simulink model "bbsr_sim"  (R2022b)
settings: Solver=VariableStepAuto  StartTime=0.0  StopTime=tmax  MaxStep=dt  RelTol=1e-3
values from neighbouring files (symbols this model uses):
  burning_rate = 1018/32.42    (= 31.4003701419)    [black_brant_vc.m]
  D0 = 1.225    [earth.m]
  fthrust = 69.4*10^3    (= 69400)    [black_brant_vc.m]
  G = 6.67430*10^-11    (= 6.6743e-11)    [bbsr_driverfile.m]
  H = 7640    [earth.m]
  mearth = 5.9722*10^24    (= 5.9722e+24)    [earth.m]
  mfuel = 1018    [black_brant_vc.m]
  mpayload = 100    [black_brant_vc.m]
  mrocket = 1261    [black_brant_vc.m]
  nozzle_area = pi*0.34^2    (= 0.363168110755)    [black_brant_vc.m]
  P0 = 1.01325*10^5    (= 101325)    [earth.m]
  pitch = 60*rad    (= 1.0471975512)    [bbsr_driverfile.m]
  r_earth = 6.3781*10^6    (= 6378100)    [earth.m]
  railheight = sin(pitch)*25    [bbsr_driverfile.m]
  v0 = 0    [bbsr_driverfile.m]
  x0 = 0    [bbsr_driverfile.m]
  y0 = 0    [bbsr_driverfile.m]
libraries: simulink x1
settings Model: Creator=mitch  LastModifiedBy=mitch
settings DataIOCC: ReturnWorkspaceOutputs=off

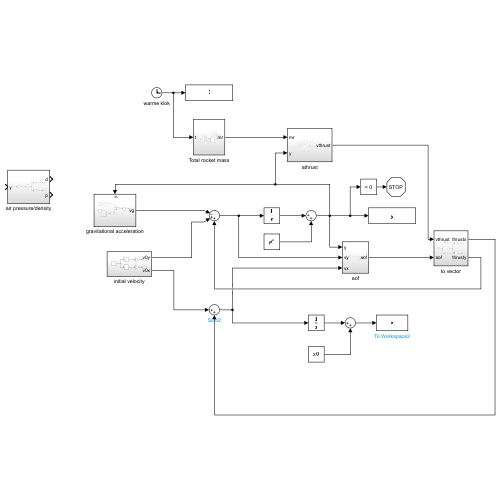
[thumbnail: Simulink's stored preview of the top-level diagram]
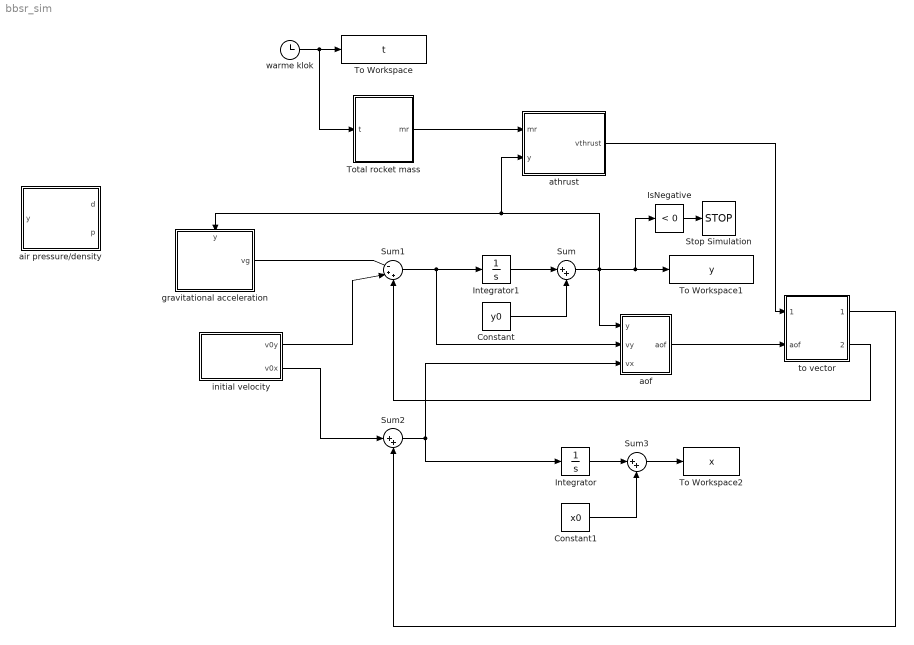
== system bbsr_sim ==
  Constant : Constant  Value=y0
  Constant1 : Constant  Value=x0
  Integrator : Integrator
  Integrator1 : Integrator
  IsNegative : simulink/Logic and Bit Operations/Compare To Zero  relop=<  OutDataTypeStr=boolean
      settings: LibrarySourceBlock=|
      | simulink/Quick Insert/Logic and Bit
      | Operations/IsNegative
  Stop Simulation : Stop
  Sum : Sum  Inputs=|++
  Sum1 : Sum  Inputs=|-++
  Sum2 : Sum  Inputs=|++
  Sum3 : Sum  Inputs=|++
  To Workspace : ToWorkspace  VariableName=t  SampleTime=-1
  To Workspace1 : ToWorkspace  VariableName=y  SampleTime=-1
  To Workspace2 : ToWorkspace  VariableName=x  SampleTime=-1
  Total rocket mass : Subsystem
  air pressure/density : Subsystem
  aof : Subsystem
  athrust : Subsystem
  gravitational acceleration : Subsystem
      settings: PortSchema="{\"entries\":[{\"content\":{\"sides\":[{\"content\":{\"connectorIds\":[]},\"type\":\"ConnectorPlacement.EquallySpacedRectSide\",\"uuid\":\"49ae1f6c-9b05-4d5e-bf5d-de0f817c918d\"},{\"content\":{\"connectorIds\":[\"Out1\"],\"side\":\"RIGHT\"},\"type\":\"ConnectorPlacement.EquallySpacedRectSide\",\"uuid\":\"2668f6bc-3456-4f0e-9125-4666e44a9436\"},{\"content\":{\"connectorIds\":[\"In1\"],\"side\":\"TOP\"},\"type\":\"ConnectorPlacement.EquallySpacedRectSide\",\"uuid\":\"db408307-21fd-484d-89bb-a4b1247c71c3\"}]},\"type\":\"ConnectorPlacement.EquallySpacedConnector\",\"uuid\":\"81d98a46-5b23-44e6-b19a-9d7581a6447a\"}],\"packageUris\":[\"http://schema.mathworks.com/mf0/Connector/R2020b\"],\"version\":\"1.0\"}"
  initial velocity : Subsystem
  to vector : Subsystem
  warme klok : Clock
  wires:
  warme klok/1 -> Total rocket mass/1(t), To Workspace/1
  Total rocket mass/1(mr) -> athrust/1(mr)
  Integrator1/1 -> Sum/1
  Sum/1 -> aof/1(y), athrust/2(y), gravitational acceleration/1(y), IsNegative/1, To Workspace1/1
  Constant/1 -> Sum/2
  gravitational acceleration/1(vg) -> Sum1/1
  Sum1/1 -> aof/2(vy), Integrator1/1
  initial velocity/1(v0y) -> Sum1/2
  athrust/1(vthrust) -> to vector/1(vthrust)
  aof/1(aof) -> to vector/2(aof)
  to vector/2(thrusty) -> Sum1/3
  initial velocity/2(v0x) -> Sum2/1
  to vector/1(thrustx) -> Sum2/2
  Sum2/1 -> aof/3(vx), Integrator/1
  Integrator/1 -> Sum3/1
  Sum3/1 -> To Workspace2/1
  Constant1/1 -> Sum3/2
  IsNegative/1 -> Stop Simulation/1

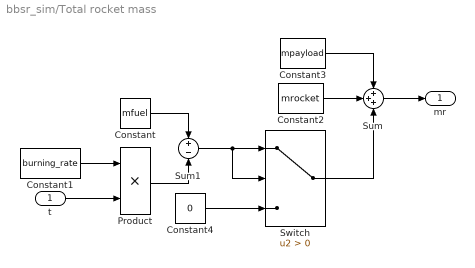
== system bbsr_sim/Total rocket mass ==
  t : Inport
  Constant : Constant  Value=mfuel
  Constant1 : Constant  Value=burning_rate
  Constant2 : Constant  Value=mrocket
  Constant3 : Constant  Value=mpayload
  Constant4 : Constant  Value=0
  Product : Product
  Sum : Sum  Inputs=+++
  Sum1 : Sum  Inputs=+-
  Switch : Switch  Criteria=u2 > Threshold  SaturateOnIntegerOverflow=off  InputSameDT=off
  mr : Outport
  wires:
  Constant3/1 -> Sum/1
  Constant1/1 -> Product/1
  t/1 -> Product/2
  Constant2/1 -> Sum/2
  Constant4/1 -> Switch/3
  Constant/1 -> Sum1/1
  Sum1/1 -> Switch/1, Switch/2
  Product/1 -> Sum1/2
  Switch/1 -> Sum/3
  Sum/1 -> mr/1

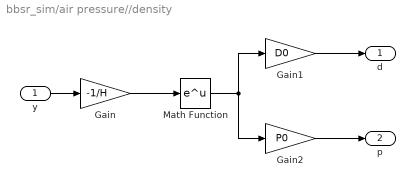
== system bbsr_sim/air pressure//density ==
  y : Inport
  Gain : Gain  Gain=-1/H
  Gain1 : Gain  Gain=D0
  Gain2 : Gain  Gain=P0
  Math Function : Math
  d : Outport
  p : Outport  Port=2
  wires:
  y/1 -> Gain/1
  Gain/1 -> Math Function/1
  Math Function/1 -> Gain2/1, Gain1/1
  Gain1/1 -> d/1
  Gain2/1 -> p/1

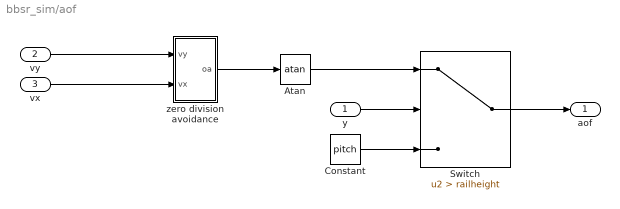
== system bbsr_sim/aof ==
  y : Inport
  vy : Inport  Port=2
  vx : Inport  Port=3
  Atan : Trigonometry  Operator=atan
  Constant : Constant  Value=pitch
  Switch : Switch  Criteria=u2 > Threshold  Threshold=railheight  SaturateOnIntegerOverflow=off  InputSameDT=off
  zero division avoidance : Subsystem
  aof : Outport
  wires:
  y/1 -> Switch/2
  Constant/1 -> Switch/3
  vy/1 -> zero division avoidance/1(vy)
  vx/1 -> zero division avoidance/2(vx)
  zero division avoidance/1(oa) -> Atan/1
  Atan/1 -> Switch/1
  Switch/1 -> aof/1

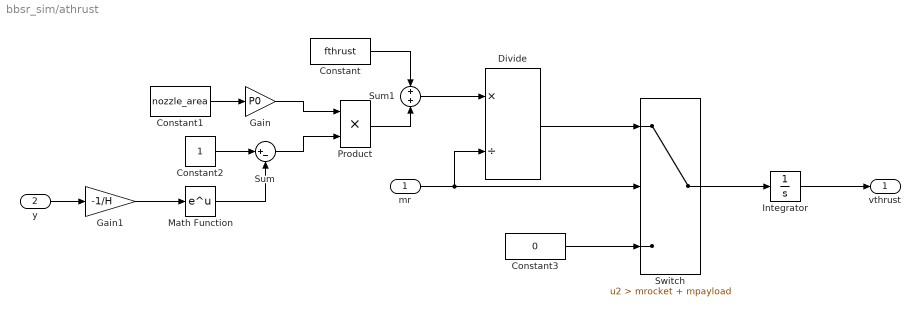
== system bbsr_sim/athrust ==
  mr : Inport
  y : Inport  Port=2
  Constant : Constant  Value=fthrust
  Constant1 : Constant  Value=nozzle_area
  Constant2 : Constant
  Constant3 : Constant  Value=0
  Divide : Product  Inputs=*/
  Gain : Gain  Gain=P0
  Gain1 : Gain  Gain=-1/H
  Integrator : Integrator
  Math Function : Math
  Product : Product
  Sum : Sum  Inputs=|+-
  Sum1 : Sum
  Switch : Switch  Criteria=u2 > Threshold  Threshold=mrocket + mpayload  SaturateOnIntegerOverflow=off  InputSameDT=off
  vthrust : Outport
  wires:
  Math Function/1 -> Sum/2
  Constant1/1 -> Gain/1
  Gain1/1 -> Math Function/1
  Constant2/1 -> Sum/1
  y/1 -> Gain1/1
  Gain/1 -> Product/1
  Sum/1 -> Product/2
  Product/1 -> Sum1/2
  Constant/1 -> Sum1/1
  Sum1/1 -> Divide/1
  mr/1 -> Divide/2, Switch/2
  Divide/1 -> Switch/1
  Constant3/1 -> Switch/3
  Switch/1 -> Integrator/1
  Integrator/1 -> vthrust/1

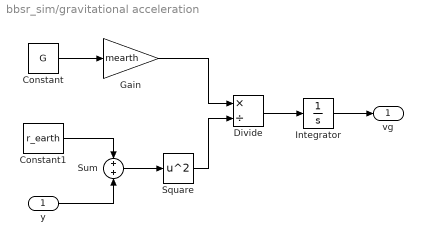
== system bbsr_sim/gravitational acceleration ==
  y : Inport
  Constant : Constant  Value=G
  Constant1 : Constant  Value=r_earth
  Divide : Product  Inputs=*/
  Gain : Gain  Gain=mearth
  Integrator : Integrator
  Square : Math  Operator=square
  Sum : Sum
  vg : Outport
  wires:
  y/1 -> Sum/2
  Constant1/1 -> Sum/1
  Constant/1 -> Gain/1
  Gain/1 -> Divide/1
  Sum/1 -> Square/1
  Square/1 -> Divide/2
  Integrator/1 -> vg/1
  Divide/1 -> Integrator/1

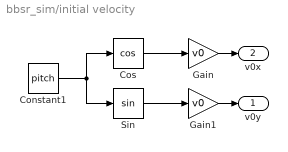
== system bbsr_sim/initial velocity ==
  Constant1 : Constant  Value=pitch
  Cos : Trigonometry  Operator=cos
  Gain : Gain  Gain=v0
  Gain1 : Gain  Gain=v0
  Sin : Trigonometry
  v0y : Outport
  v0x : Outport  Port=2
  wires:
  Constant1/1 -> Cos/1, Sin/1
  Cos/1 -> Gain/1
  Sin/1 -> Gain1/1
  Gain1/1 -> v0y/1
  Gain/1 -> v0x/1

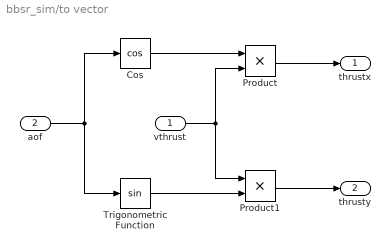
== system bbsr_sim/to vector ==
  vthrust : Inport
  aof : Inport  Port=2
  Cos : Trigonometry  Operator=cos
  Product : Product
  Product1 : Product
  Trigonometric Function : Trigonometry
  thrustx : Outport
  thrusty : Outport  Port=2
  wires:
  Cos/1 -> Product/1
  Trigonometric Function/1 -> Product1/2
  aof/1 -> Trigonometric Function/1, Cos/1
  vthrust/1 -> Product1/1, Product/2
  Product/1 -> thrustx/1
  Product1/1 -> thrusty/1

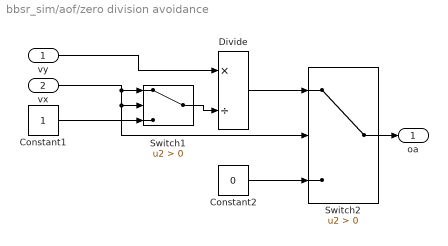
== system bbsr_sim/aof/zero division avoidance ==
  vy : Inport
  vx : Inport  Port=2
  Constant1 : Constant
  Constant2 : Constant  Value=0
  Divide : Product  Inputs=*/
  Switch1 : Switch  Criteria=u2 > Threshold  SaturateOnIntegerOverflow=off  InputSameDT=off
  Switch2 : Switch  Criteria=u2 > Threshold  SaturateOnIntegerOverflow=off  InputSameDT=off
  oa : Outport
  wires:
  vx/1 -> Switch1/2, Switch2/2, Switch1/1
  Switch1/1 -> Divide/2
  Constant2/1 -> Switch2/3
  vy/1 -> Divide/1
  Divide/1 -> Switch2/1
  Constant1/1 -> Switch1/3
  Switch2/1 -> oa/1
